simulink model "mass_spring_damper"  (R2025b)
settings: Solver=ode45  StartTime=0.0  StopTime=100  MaxStep=0.01  RelTol=1e-3  EnableMultiTasking=on
settings Model: Creator=nike  LastModifiedBy=ZBook Fury
settings SolverCC: AlgebraicLoopSolver=TrustRegion
settings DataIOCC: LimitDataPoints=on  SaveFormat=Array  SignalLoggingSaveFormat=ModelDataLogs  ReturnWorkspaceOutputs=off
settings OptimizationCC: ExpressionDepthLimit=2147483647.0  LifeSpan=inf
settings DebuggingCC: UnderspecifiedInitializationDetection=Classic  MergeDetectMultiDrivingBlocksExec=none  SolverPrmCheckMsg=warning  FcnCallInpInsideContextMsg=warning  UnconnectedInputMsg=warning  UnconnectedOutputMsg=warning  UnconnectedLineMsg=warning  StateNameClashWarn=warning  SFUnexpectedBacktrackingDiag=warning  SFNoUnconditionalDefaultTransitionDiag=warning  SFExecutionAtInitializationDiag=none  ArithmeticOperatorsInVariantConditions=warning
settings HardwareCC: ProdBitPerPointer=32.0  ProdBitPerSizeT=32.0  ProdBitPerPtrDiffT=32.0  ProdLargestAtomicFloat=None  ProdIntDivRoundTo=Undefined  ProdEndianess=Unspecified  ProdWordSize=32.0  ProdHWDeviceType=32-bit Generic
settings ModelReferenceCC: PropagateSignalLabelsOutOfModel=off
settings SFSimCC: SimUseLocalCustomCode=off  CustomCodeUndefinedFunction=UseInterfaceOnly
settings RTWCC: RTWUseLocalCustomCode=off  GPUComputeCapability=3.5
settings CodeAppCC: StateflowObjectComments=on
settings GRTTargetCC: TargetLangStandard=C89/C90 (ANSI)  CombineOutputUpdateFcns=off  GRTInterface=on
settings ConfigComp: CovMetricSettings=dw  CovSaveCumulativeToWorkspaceVar=on  CovSaveSingleToWorkspaceVar=on  CovExternalEMLEnable=off

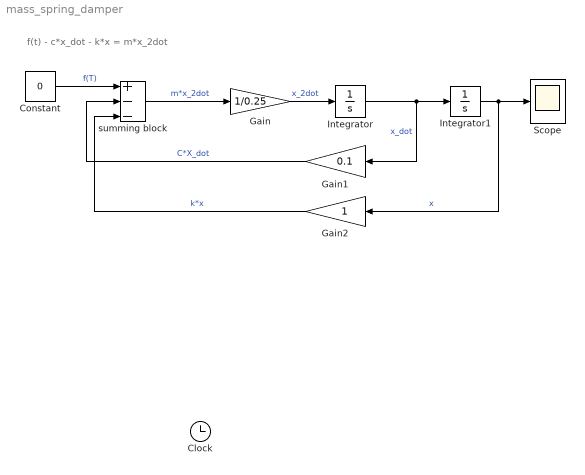
== system mass_spring_damper ==
  note: f(t) - c*x_dot - k*x = m*x_2dot
  Constant : Constant  Value=0
  Gain : Gain  Gain=1/0.25
  Gain1 : Gain  Gain=0.1
  Gain2 : Gain
  Integrator : Integrator
  Integrator1 : Integrator  InitialCondition=10
  Scope : Scope
      settings: ActiveDisplayYMinimum=-9.4536595613953249  ActiveDisplayYMaximum=12.161517729043926
  summing block : Sum  Inputs=+--
  Clock : Clock
      settings: IOType=siggen
  wires:
  Constant/1 -> summing block/1  "f(T)"
  Gain1/1 -> summing block/2  "C*X_dot"
  summing block/1 -> Gain/1  "m*x_2dot"
  Gain/1 -> Integrator/1  "x_2dot"
  Integrator1/1 -> Scope/1, Gain2/1  "x"
  Integrator/1 -> Integrator1/1, Gain1/1  "x_dot"
  Gain2/1 -> summing block/3  "k*x"
